simulink model "discrete_PID_2_1_1_5_b"  (R2024b)
settings: Solver=ode5  StartTime=0.0  StopTime=10  FixedStep=10e-6  RelTol=1e-3
values from neighbouring files (symbols this model uses):
  T = T2    (= 0.01)    [Tustin.m]
undefined symbols (not defined in the file or in its folder): daq, DiscIntNeverNeededParam, drv, gbox, kd, ki, kp, mld, mot, rads2rpm, sens, tl, u_bar_max
settings Model: Creator=Enrico  LastModifiedBy=farin

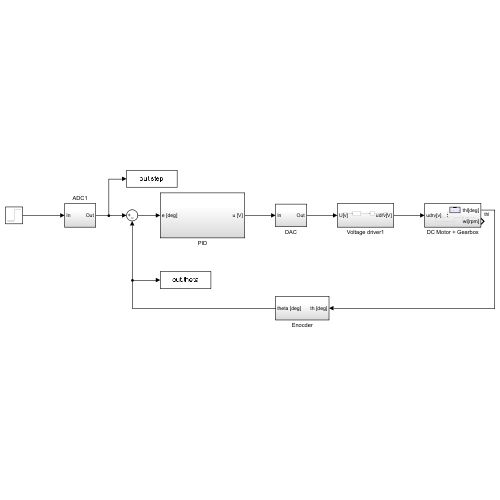
[thumbnail: Simulink's stored preview of the top-level diagram]
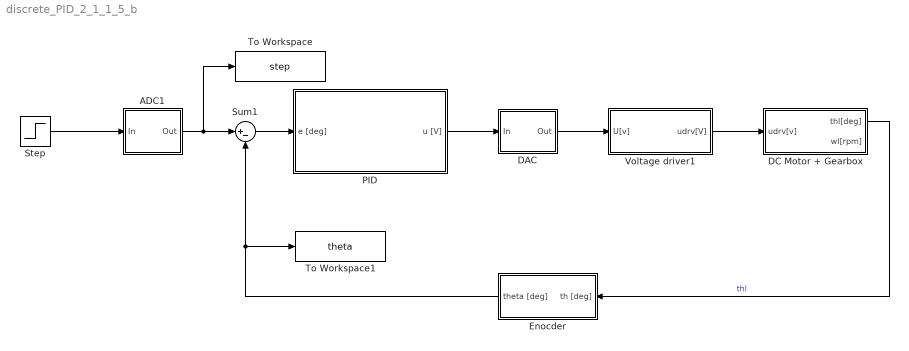
== system discrete_PID_2_1_1_5_b ==
  ADC1 : Subsystem
  DAC : Subsystem
  DC Motor + Gearbox : Subsystem
  Enocder : Subsystem
  PID : Subsystem
  Step : Step  After=50  SampleTime=0
  Sum1 : Sum  Inputs=|+-
  To Workspace : ToWorkspace  VariableName=step  SaveFormat=Structure With Time  SampleTime=-1
  To Workspace1 : ToWorkspace  VariableName=theta  SaveFormat=Structure With Time  SampleTime=-1
  Voltage driver1 : Subsystem
  wires:
  ADC1/1(Out) -> To Workspace/1, Sum1/1
  Sum1/1 -> PID/1(e [deg])
  PID/1(u [V]) -> DAC/1(In)
  DAC/1(Out) -> Voltage driver1/1(U[v])
  Voltage driver1/1(udrv[V]) -> DC Motor + Gearbox/1(udrv[v])
  DC Motor + Gearbox/1(thl[deg]) -> Enocder/1(th [deg])  "thl"
  Step/1 -> ADC1/1(In)
  Enocder/1(theta [deg]) -> Sum1/2, To Workspace1/1

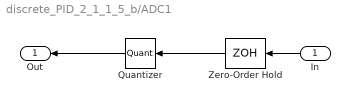
== system discrete_PID_2_1_1_5_b/ADC1 ==
  In : Inport
  Quantizer : Quantizer  QuantizationInterval=daq.adc.q
  Zero-Order Hold : ZeroOrderHold  SampleTime=T
  Out : Outport
  wires:
  Quantizer/1 -> Out/1
  In/1 -> Zero-Order Hold/1
  Zero-Order Hold/1 -> Quantizer/1

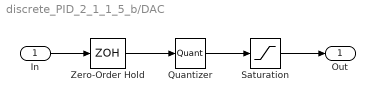
== system discrete_PID_2_1_1_5_b/DAC ==
  In : Inport
  Quantizer : Quantizer  QuantizationInterval=daq.dac.q
  Saturation : Saturate  UpperLimit=daq.dac.fs  LowerLimit=-daq.dac.fs
  Zero-Order Hold : ZeroOrderHold  SampleTime=T
  Out : Outport
  wires:
  Quantizer/1 -> Saturation/1
  In/1 -> Zero-Order Hold/1
  Zero-Order Hold/1 -> Quantizer/1
  Saturation/1 -> Out/1

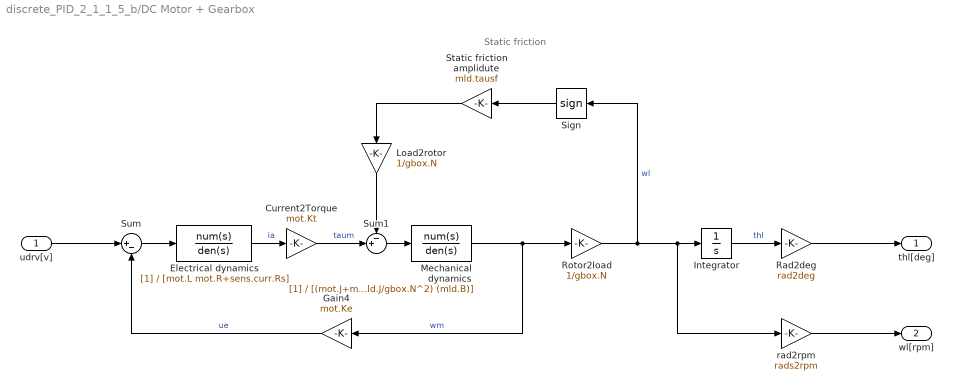
== system discrete_PID_2_1_1_5_b/DC Motor + Gearbox ==
  note: Static friction
  udrv[v] : Inport
  " Sign" : Signum  ZeroCross=off
  Current2Torque : Gain  Gain=mot.Kt
  Electrical dynamics : TransferFcn  Denominator=[mot.L mot.R+sens.curr.Rs]
  Gain4 : Gain  Gain=mot.Ke
  Integrator : Integrator
  Load2rotor : Gain  Gain=1/gbox.N
  Mechanical dynamics : TransferFcn  Denominator=[(mot.J+mld.J/gbox.N^2) (mld.B)]
  Rad2deg : Gain  Gain=rad2deg
  Rotor2load : Gain  Gain=1/gbox.N
  Static friction amplidute : Gain  Gain=mld.tausf
  Sum : Sum  Inputs=|+-
  Sum1 : Sum  Inputs=-+|
  rad2rpm : Gain  Gain=rads2rpm
  thl[deg] : Outport
  wl[rpm] : Outport  Port=2
  wires:
  udrv[v]/1 -> Sum/1
  Sum/1 -> Electrical dynamics/1
  Electrical dynamics/1 -> Current2Torque/1  "ia"
  Current2Torque/1 -> Sum1/2  "taum"
  Load2rotor/1 -> Sum1/1
  " Sign"/1 -> Static friction amplidute/1
  Static friction amplidute/1 -> Load2rotor/1
  Sum1/1 -> Mechanical dynamics/1
  Mechanical dynamics/1 -> Gain4/1, Rotor2load/1  "wm"
  Gain4/1 -> Sum/2  "ue"
  Rad2deg/1 -> thl[deg]/1
  rad2rpm/1 -> wl[rpm]/1
  Integrator/1 -> Rad2deg/1  "thl"
  Rotor2load/1 -> " Sign"/1, rad2rpm/1, Integrator/1  "wl"

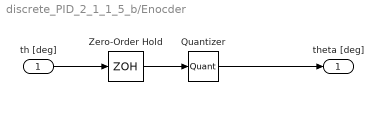
== system discrete_PID_2_1_1_5_b/Enocder ==
  th [deg] : Inport
  Quantizer : Quantizer  QuantizationInterval=sens.enc.pulse2deg
  Zero-Order Hold : ZeroOrderHold  SampleTime=T
  theta [deg] : Outport
  wires:
  th [deg]/1 -> Zero-Order Hold/1
  Zero-Order Hold/1 -> Quantizer/1
  Quantizer/1 -> theta [deg]/1

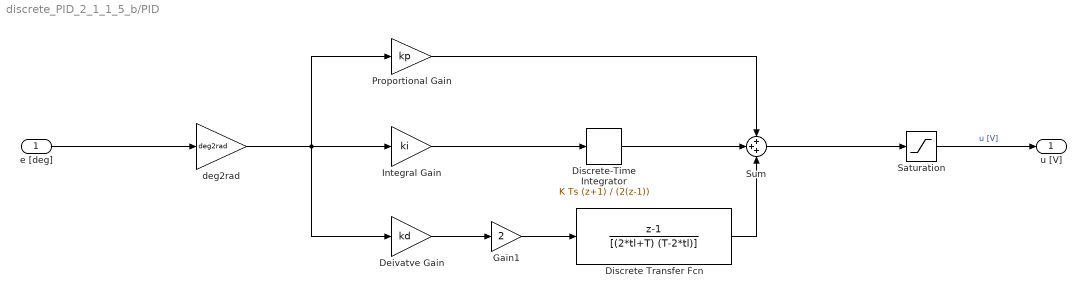
== system discrete_PID_2_1_1_5_b/PID ==
  e [deg] : Inport
  Deivatve Gain : Gain  Gain=kd
  Discrete Transfer Fcn : DiscreteTransferFcn  Numerator=[1 -1]  Denominator=[(2*tl+T) (T-2*tl)]
  Discrete-Time Integrator : DiscreteIntegrator  IntegratorMethod=Integration: Trapezoidal  gainval=1  SampleTime=T  ICPrevOutput=DiscIntNeverNeededParam  ICPrevScaledInput=DiscIntNeverNeededParam
  Gain1 : Gain  Gain=2
  Integral Gain : Gain  Gain=ki
  Proportional Gain : Gain  Gain=kp
  "Saturation " : Saturate  UpperLimit=u_bar_max  LowerLimit=-u_bar_max
  Sum : Sum  Inputs=+++
  deg2rad : Gain  Gain=deg2rad
  u [V] : Outport
  wires:
  e [deg]/1 -> deg2rad/1
  "Saturation "/1 -> u [V]/1  "u [V]"
  deg2rad/1 -> Deivatve Gain/1, Proportional Gain/1, Integral Gain/1
  Discrete Transfer Fcn/1 -> Sum/3
  Proportional Gain/1 -> Sum/1
  Sum/1 -> "Saturation "/1
  Integral Gain/1 -> Discrete-Time Integrator/1
  Discrete-Time Integrator/1 -> Sum/2
  Gain1/1 -> Discrete Transfer Fcn/1
  Deivatve Gain/1 -> Gain1/1

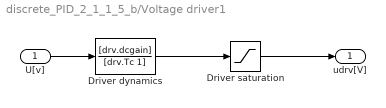
== system discrete_PID_2_1_1_5_b/Voltage driver1 ==
  U[v] : Inport
  Driver dynamics : TransferFcn  Numerator=[drv.dcgain]  Denominator=[drv.Tc 1]
  Driver saturation : Saturate  UpperLimit=12  LowerLimit=-12
  udrv[V] : Outport
  wires:
  U[v]/1 -> Driver dynamics/1
  Driver dynamics/1 -> Driver saturation/1
  Driver saturation/1 -> udrv[V]/1
